simulink model "Copy_of_ModeStatAndRsp"  (R2018b)
settings: Solver=FixedStepDiscrete  StartTime=0.0  StopTime=10.0  FixedStep=0.01  RelTol=1e-3
undefined symbols (not defined in the file): c_RecvL, c_RecvLR, c_RecvR, IfVeSMSeStNumConfig, KeSMSbMdChime2Enable_Val, KeSMSbSRSPosNumConfig_Val, KeSMSuChmReqDurnTm_Val, KeSMSuChmReqIntlTm_Val, KeSMSuRspStatHldTm_Val, MdRspLocal1, MdTp1, ModeNum, PowerMode1, SrcReqTp1, srsconvert
libraries: RspLib x47, simulink x1
(part 4 of 8)

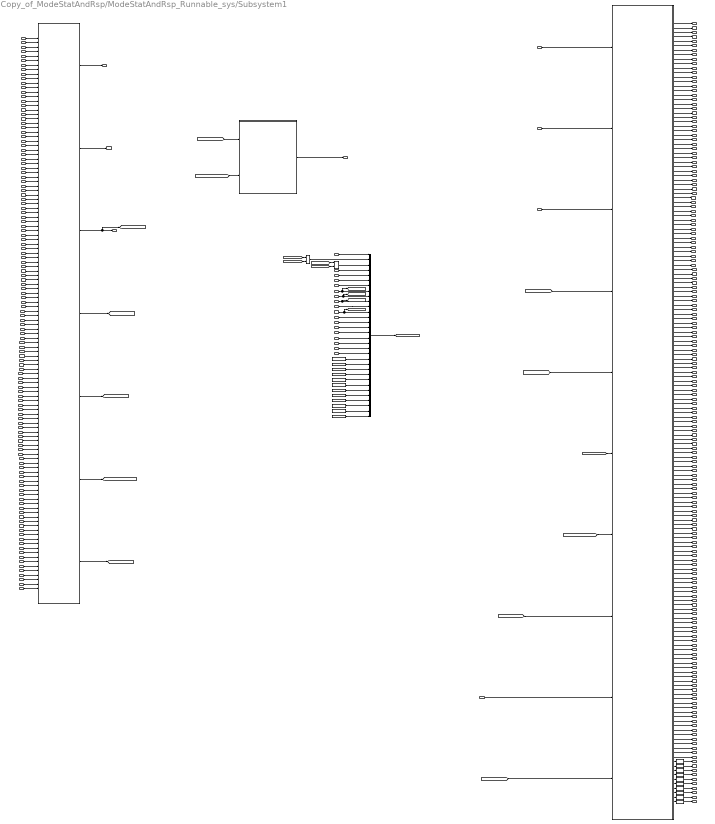
== system Copy_of_ModeStatAndRsp/ModeStatAndRsp_Runnable_sys/Subsystem1 ==
  acsExtMdReq : Inport
  acsEntyMdReq : Inport  Port=2
  LtVipMdReq : Inport  Port=3
  RtVipMdReq : Inport  Port=4
  AllVipMdReq : Inport  Port=5
  LtLugMdReq : Inport  Port=6
  RtLugMdReq : Inport  Port=7
  AllLugMdReq : Inport  Port=8
  LtRcvyMdReq : Inport  Port=9
  RtRcvyMdReq : Inport  Port=10
  CommCond : Inport  Port=11
  CommExitCond : Inport  Port=12
  CommExitCondwithSpeed : Inport  Port=13
  isAcsMdEntryDoneOK : Inport  Port=14
  isAcsMdExtDoneOK : Inport  Port=15
  isLfLugDoneOK : Inport  Port=16
  isLfRecoveryDoneOK : Inport  Port=17
  isLfVipDoneOK : Inport  Port=18
  isRtLugDoneOK : Inport  Port=19
  isRtRecoveryDoneOK : Inport  Port=20
  isRtVipDoneOK : Inport  Port=21
  isAcsMdEntryDoneFailed : Inport  Port=22
  isAcsMdExtDoneFailed : Inport  Port=23
  isLfLugDoneFailed : Inport  Port=24
  isLfRecoveryDoneFailed : Inport  Port=25
  isLfVipDoneFailed : Inport  Port=26
  isRtLugDoneFailed : Inport  Port=27
  isRtRecoveryDoneFailed : Inport  Port=28
  isRtVipDoneFailed : Inport  Port=29
  SwIntAcsEnty : Inport  Port=30
  SwIntAcsExt : Inport  Port=31
  SwIntLfVip : Inport  Port=32
  SwIntRtVip : Inport  Port=33
  SwIntLfLug : Inport  Port=34
  SwIntRtLug : Inport  Port=35
  SwIntLfRcvy : Inport  Port=36
  SwIntRtRcvy : Inport  Port=37
  SwIntAllLug : Inport  Port=38
  SoftIntAcsExt : Inport  Port=39
  SoftIntAcsEnty : Inport  Port=40
  SoftIntLfVip : Inport  Port=41
  SoftIntRtVip : Inport  Port=42
  SoftIntLfLug : Inport  Port=43
  SoftIntRtLug : Inport  Port=44
  SoftIntLfRcvy : Inport  Port=45
  SoftIntRtRcvy : Inport  Port=46
  SoftIntAllVip : Inport  Port=47
  SoftIntAllLug : Inport  Port=48
  acsExtMdSrcTp : Inport  Port=49
  acsEntyMdSrcTp : Inport  Port=50
  LtVipSrcReqTp : Inport  Port=51
  RtVipSrcReqTp : Inport  Port=52
  LtLugSrcReqTp : Inport  Port=53
  RtLugSrcReqTp : Inport  Port=54
  LtRcvySrcReqTp : Inport  Port=55
  RtRcvySrcReqTp : Inport  Port=56
  PwrMdChked : Inport  Port=57
  isLfLugArrivedAtTargetPos : Inport  Port=58
  isRtLugArrivedAtTargetPos : Inport  Port=59
  isLfVipArrivedAtTargetPos : Inport  Port=60
  isRtVipArrivedAtTargetPos : Inport  Port=61
  isAcsMdEntryArrivedAtTargetPos : Inport  Port=62
  isAcsMdExtArrivedAtTargetPos : Inport  Port=63
  isLfRecoveryArrivedAtTargetPos : Inport  Port=64
  isRtRecoveryArrivedAtTargetPos : Inport  Port=65
  IfVeSMSuChmMgrStat_Val_read : Inport  Port=66
  KeSMSuRspStatHldTm_Val : Inport  Port=67
  AllLugSrcReqTp_Val : Inport  Port=68
  StNumConfig : Inport  Port=69
  isAcsMdINTMAtTargetPos : Inport  Port=70
  isAcsMdFamlyLAtTargetPos : Inport  Port=71
  isAcsMdFamlyRAtTargetPos : Inport  Port=72
  isLyLArrivedAtTargetPos : Inport  Port=73
  isLyRArrivedAtTargetPos : Inport  Port=74
  isINTMDoneOK : Inport  Port=75
  isFamlyLDoneOK : Inport  Port=76
  isFamlyRDoneOK : Inport  Port=77
  isLfLyDoneOK : Inport  Port=78
  isRtLyDoneOK : Inport  Port=79
  isINTMDoneFailed : Inport  Port=80
  isFamlyLDoneFailed : Inport  Port=81
  isFamlyRDoneFailed : Inport  Port=82
  isLfLyDoneFailed : Inport  Port=83
  isRtLyDoneFailed : Inport  Port=84
  INTMMdReq_Val_read : Inport  Port=85
  INTMSrcReqTp_Val_read : Inport  Port=86
  LfFamlyReq_Val_read : Inport  Port=87
  LfFamlySrcReqTp_Val_read : Inport  Port=88
  LfLyMdReq_Val_read : Inport  Port=89
  LfLySrcReqTp_Val_read : Inport  Port=90
  RtFamlyMdReq_Val_read : Inport  Port=91
  RtFamlySrcReqTp_Val_read : Inport  Port=92
  RtLyMdReq_Val_read : Inport  Port=93
  RtLySrcReqTp_Val_read : Inport  Port=94
  SoftIntINTM_Val_read : Inport  Port=95
  SoftIntLfFamly_Val_read : Inport  Port=96
  SoftIntLfLy_Val_read : Inport  Port=97
  SoftIntRtFamly_Val_read : Inport  Port=98
  SoftIntRtLy_Val_read : Inport  Port=99
  SwIntINTM_Val_read : Inport  Port=100
  SwIntLfFamly_Val_read : Inport  Port=101
  SwIntLfLy_Val_read : Inport  Port=102
  SwIntRtFamly_Val_read : Inport  Port=103
  SwIntRtLy_Val_read : Inport  Port=104
  PosArray_Val_read : Inport  Port=105
  AllVipSrcReqTp_Val_read : Inport  Port=106
  LugMdLtAvl_Val_read : Inport  Port=107
  LugMdRtAvl_Val_read : Inport  Port=108
  VipMdLtAvl_Val_read : Inport  Port=109
  VipMdRtAvl_Val_read : Inport  Port=110
  SwIntAllVip_Val_read : Inport  Port=111
  IntimacyRtMdReq_Val_read : Inport  Port=112
  IntimacyRtMdSrcTp_Val_read : Inport  Port=113
  isINTMRArrivedAtTargetPos_Val_read : Inport  Port=114
  isINTMRDoneFailed_Val_read : Inport  Port=115
  isINTMRDoneOK_Val_read : Inport  Port=116
  isLgrstCloseLArrivedAtTargetPos_Val_read : Inport  Port=117
  isLgrstCloseLDoneFailed_Val_read : Inport  Port=118
  isLgrstCloseLDoneOK_Val_read : Inport  Port=119
  isLgrstCloseRArrivedAtTargetPos_Val_read : Inport  Port=120
  isLgrstCloseRDoneFailed_Val_read : Inport  Port=121
  isLgrstCloseRDoneOK_Val_read : Inport  Port=122
  isLgrstOpenLArrivedAtTargetPos_Val_read : Inport  Port=123
  isLgrstOpenLDoneFailed_Val_read : Inport  Port=124
  isLgrstOpenLDoneOK_Val_read : Inport  Port=125
  isLgrstOpenRArrivedAtTargetPos_Val_read : Inport  Port=126
  isLgrstOpenRDoneFailed_Val_read : Inport  Port=127
  isLgrstOpenRDoneOK_Val_read : Inport  Port=128
  LgrstCloseLtMdReq_Val_read : Inport  Port=129
  LgrstCloseLtSrcReqTp_Val_read : Inport  Port=130
  LgrstCloseRtMdReq_Val_read : Inport  Port=131
  LgrstCloseRtSrcReqTp_Val_read : Inport  Port=132
  LgrstOpenLtMdReq_Val_read : Inport  Port=133
  LgrstOpenLtSrcReqTp_Val_read : Inport  Port=134
  LgrstOpenRtMdReq_Val_read : Inport  Port=135
  LgrstOpenRtSrcReqTp_Val_read : Inport  Port=136
  SoftIntIntimacyRt_Val_read : Inport  Port=137
  SoftIntLgrstCloseLt_Val_read : Inport  Port=138
  SoftIntLgrstCloseRt_Val_read : Inport  Port=139
  SoftIntLgrstOpenLt_Val_read : Inport  Port=140
  SoftIntLgrstOpenRt_Val_read : Inport  Port=141
  SwIntIntimacyRt_Val_read : Inport  Port=142
  SwIntLgrstCloseLt_Val_read : Inport  Port=143
  SwIntLgrstCloseRt_Val_read : Inport  Port=144
  SwIntLgrstOpenLt_Val_read : Inport  Port=145
  SwIntLgrstOpenRt_Val_read : Inport  Port=146
  AND : Logic  AllPortsSameDT=off  OutDataTypeStr=boolean
  AND1 : Logic  AllPortsSameDT=off  OutDataTypeStr=boolean
  Bus Creator2 : BusCreator  Inputs=32
  Constant{39..50} (12 alike) : Constant  Value=0  OutDataTypeStr=boolean
  Data Type Conversion{,1..9} (10 alike) : DataTypeConversion  OutDataTypeStr=uint8
  FeedbackModeStatAndRsp : Subsystem
  SRSModeCheck : Subsystem
  Subsystem : Subsystem
  oModeState : Outport
  IfVeSMSeStPassCmprtMdCrtMdStat_Val_write : Outport  Port=2
  IfVeSMSeStPassCmprtMdHMIDisCmdSrv_Val_write : Outport  Port=3  VectorParamsAs1DForOutWhenUnconnected=on
  ModeSrcTpLt : Outport  Port=4  VectorParamsAs1DForOutWhenUnconnected=on
  IfVeSMSeStPassCmprtMdNoti2ChmEvntStat_Val_write : Outport  Port=5  VectorParamsAs1DForOutWhenUnconnected=on
  SRSCrtMdIndTyp_67_2_Val_write : Outport  Port=6  VectorParamsAs1DForOutWhenUnconnected=on
  ModeState32 : Outport  Port=7  VectorParamsAs1DForOutWhenUnconnected=on
  SRSMode : Outport  Port=8  VectorParamsAs1DForOutWhenUnconnected=on
  StPassCmprtMd1RclRspStat : Outport  Port=9  VectorParamsAs1DForOutWhenUnconnected=on
  StPassCmprtMd2RclRspStat : Outport  Port=10  VectorParamsAs1DForOutWhenUnconnected=on
  StPassCmprtMd3RclRspStat : Outport  Port=11  VectorParamsAs1DForOutWhenUnconnected=on
  StPassCmprtMd4RclRspStat : Outport  Port=12  VectorParamsAs1DForOutWhenUnconnected=on
  StPassCmprtMd5RclRspStat : Outport  Port=13  VectorParamsAs1DForOutWhenUnconnected=on
  StPassCmprtMd6RclRspStat : Outport  Port=14  VectorParamsAs1DForOutWhenUnconnected=on
  StPassCmprtMd7RclRspStat : Outport  Port=15  VectorParamsAs1DForOutWhenUnconnected=on
  StPassCmprtMd8RclRspStat : Outport  Port=16  VectorParamsAs1DForOutWhenUnconnected=on
  StPassCmprtMd9RclRspStat : Outport  Port=17  VectorParamsAs1DForOutWhenUnconnected=on
  StPassCmprtMd10RclRspStat : Outport  Port=18  VectorParamsAs1DForOutWhenUnconnected=on
  StPassCmprtMd11RclRspStat : Outport  Port=19  VectorParamsAs1DForOutWhenUnconnected=on
  StPassCmprtMd12RclRspStat : Outport  Port=20  VectorParamsAs1DForOutWhenUnconnected=on
  StPassCmprtMd13RclRspStat : Outport  Port=21  VectorParamsAs1DForOutWhenUnconnected=on
  StPassCmprtMd14RclRspStat : Outport  Port=22  VectorParamsAs1DForOutWhenUnconnected=on
  StPassCmprtMd15RclRspStat : Outport  Port=23  VectorParamsAs1DForOutWhenUnconnected=on
  StPassCmprtMd16RclRspStat : Outport  Port=24  VectorParamsAs1DForOutWhenUnconnected=on
  StPassCmprtMd17RclRspStat : Outport  Port=25  VectorParamsAs1DForOutWhenUnconnected=on
  StPassCmprtMd18RclRspStat : Outport  Port=26  VectorParamsAs1DForOutWhenUnconnected=on
  StPassCmprtMd19RclRspStat : Outport  Port=27  VectorParamsAs1DForOutWhenUnconnected=on
  StPassCmprtMd20RclRspStat : Outport  Port=28  VectorParamsAs1DForOutWhenUnconnected=on
  StPassCmprtMd21RclRspStat : Outport  Port=29  VectorParamsAs1DForOutWhenUnconnected=on
  StPassCmprtMd22RclRspStat : Outport  Port=30  VectorParamsAs1DForOutWhenUnconnected=on
  StPassCmprtMd23RclRspStat : Outport  Port=31  VectorParamsAs1DForOutWhenUnconnected=on
  StPassCmprtMd24RclRspStat : Outport  Port=32  VectorParamsAs1DForOutWhenUnconnected=on
  StPassCmprtMd25RclRspStat : Outport  Port=33  VectorParamsAs1DForOutWhenUnconnected=on
  StPassCmprtMd26RclRspStat : Outport  Port=34  VectorParamsAs1DForOutWhenUnconnected=on
  StPassCmprtMd27RclRspStat : Outport  Port=35  VectorParamsAs1DForOutWhenUnconnected=on
  StPassCmprtMd28RclRspStat : Outport  Port=36  VectorParamsAs1DForOutWhenUnconnected=on
  StPassCmprtMd29RclRspStat : Outport  Port=37  VectorParamsAs1DForOutWhenUnconnected=on
  StPassCmprtMd30RclRspStat : Outport  Port=38  VectorParamsAs1DForOutWhenUnconnected=on
  StPassCmprtMd31RclRspStat : Outport  Port=39  VectorParamsAs1DForOutWhenUnconnected=on
  StPassCmprtMd32RclRspStat : Outport  Port=40  VectorParamsAs1DForOutWhenUnconnected=on
  StPassCmprtMd_RfCtrl_Sw_RclRspStat : Outport  Port=41  VectorParamsAs1DForOutWhenUnconnected=on
  StSrv_StMd1_Rsp : Outport  Port=42  VectorParamsAs1DForOutWhenUnconnected=on
  StSrv_StMd2_Rsp : Outport  Port=43  VectorParamsAs1DForOutWhenUnconnected=on
  StSrv_StMd3_Rsp : Outport  Port=44  VectorParamsAs1DForOutWhenUnconnected=on
  StSrv_StMd4_Rsp : Outport  Port=45  VectorParamsAs1DForOutWhenUnconnected=on
  StSrv_StMd5_Rsp : Outport  Port=46  VectorParamsAs1DForOutWhenUnconnected=on
  StSrv_StMd6_Rsp : Outport  Port=47  VectorParamsAs1DForOutWhenUnconnected=on
  StSrv_StMd7_Rsp : Outport  Port=48  VectorParamsAs1DForOutWhenUnconnected=on
  StSrv_StMd8_Rsp : Outport  Port=49  VectorParamsAs1DForOutWhenUnconnected=on
  StSrv_StMd9_Rsp : Outport  Port=50  VectorParamsAs1DForOutWhenUnconnected=on
  StSrv_StMd10_Rsp : Outport  Port=51  VectorParamsAs1DForOutWhenUnconnected=on
  StSrv_StMd11_Rsp : Outport  Port=52  VectorParamsAs1DForOutWhenUnconnected=on
  StSrv_StMd12_Rsp : Outport  Port=53  VectorParamsAs1DForOutWhenUnconnected=on
  StSrv_StMd13_Rsp : Outport  Port=54  VectorParamsAs1DForOutWhenUnconnected=on
  StSrv_StMd14_Rsp : Outport  Port=55  VectorParamsAs1DForOutWhenUnconnected=on
  StSrv_StMd15_Rsp : Outport  Port=56  VectorParamsAs1DForOutWhenUnconnected=on
  StSrv_StMd16_Rsp : Outport  Port=57  VectorParamsAs1DForOutWhenUnconnected=on
  StSrv_StMd17_Rsp : Outport  Port=58  VectorParamsAs1DForOutWhenUnconnected=on
  StSrv_StMd18_Rsp : Outport  Port=59  VectorParamsAs1DForOutWhenUnconnected=on
  StSrv_StMd19_Rsp : Outport  Port=60  VectorParamsAs1DForOutWhenUnconnected=on
  StSrv_StMd20_Rsp : Outport  Port=61  VectorParamsAs1DForOutWhenUnconnected=on
  StSrv_StMd21_Rsp : Outport  Port=62  VectorParamsAs1DForOutWhenUnconnected=on
  StSrv_StMd22_Rsp : Outport  Port=63  VectorParamsAs1DForOutWhenUnconnected=on
  StSrv_StMd23_Rsp : Outport  Port=64  VectorParamsAs1DForOutWhenUnconnected=on
  StSrv_StMd24_Rsp : Outport  Port=65  VectorParamsAs1DForOutWhenUnconnected=on
  StSrv_StMd25_Rsp : Outport  Port=66  VectorParamsAs1DForOutWhenUnconnected=on
  StSrv_StMd26_Rsp : Outport  Port=67  VectorParamsAs1DForOutWhenUnconnected=on
  StSrv_StMd27_Rsp : Outport  Port=68  VectorParamsAs1DForOutWhenUnconnected=on
  StSrv_StMd28_Rsp : Outport  Port=69  VectorParamsAs1DForOutWhenUnconnected=on
  StSrv_StMd29_Rsp : Outport  Port=70  VectorParamsAs1DForOutWhenUnconnected=on
  StSrv_StMd30_Rsp : Outport  Port=71  VectorParamsAs1DForOutWhenUnconnected=on
  StSrv_StMd31_Rsp : Outport  Port=72  VectorParamsAs1DForOutWhenUnconnected=on
  StSrv_StMd32_Rsp : Outport  Port=73  VectorParamsAs1DForOutWhenUnconnected=on
  HMI_2L_StMd1_Rsp : Outport  Port=74  VectorParamsAs1DForOutWhenUnconnected=on
  HMI_2L_StMd2_Rsp : Outport  Port=75  VectorParamsAs1DForOutWhenUnconnected=on
  HMI_2L_StMd3_Rsp : Outport  Port=76  VectorParamsAs1DForOutWhenUnconnected=on
  HMI_2L_StMd4_Rsp : Outport  Port=77  VectorParamsAs1DForOutWhenUnconnected=on
  HMI_2L_StMd5_Rsp : Outport  Port=78  VectorParamsAs1DForOutWhenUnconnected=on
  HMI_2L_StMd6_Rsp : Outport  Port=79  VectorParamsAs1DForOutWhenUnconnected=on
  HMI_2L_StMd7_Rsp : Outport  Port=80  VectorParamsAs1DForOutWhenUnconnected=on
  HMI_2L_StMd8_Rsp : Outport  Port=81  VectorParamsAs1DForOutWhenUnconnected=on
  HMI_2L_StMd9_Rsp : Outport  Port=82  VectorParamsAs1DForOutWhenUnconnected=on
  HMI_2L_StMd10_Rsp : Outport  Port=83  VectorParamsAs1DForOutWhenUnconnected=on
  HMI_2L_StMd11_Rsp : Outport  Port=84  VectorParamsAs1DForOutWhenUnconnected=on
  HMI_2L_StMd12_Rsp : Outport  Port=85  VectorParamsAs1DForOutWhenUnconnected=on
  HMI_2L_StMd13_Rsp : Outport  Port=86  VectorParamsAs1DForOutWhenUnconnected=on
  HMI_2L_StMd14_Rsp : Outport  Port=87  VectorParamsAs1DForOutWhenUnconnected=on
  HMI_2L_StMd15_Rsp : Outport  Port=88  VectorParamsAs1DForOutWhenUnconnected=on
  HMI_2L_StMd16_Rsp : Outport  Port=89  VectorParamsAs1DForOutWhenUnconnected=on
  HMI_2L_StMd17_Rsp : Outport  Port=90  VectorParamsAs1DForOutWhenUnconnected=on
  HMI_2L_StMd18_Rsp : Outport  Port=91  VectorParamsAs1DForOutWhenUnconnected=on
  HMI_2L_StMd19_Rsp : Outport  Port=92  VectorParamsAs1DForOutWhenUnconnected=on
  HMI_2L_StMd20_Rsp : Outport  Port=93  VectorParamsAs1DForOutWhenUnconnected=on
  HMI_2L_StMd21_Rsp : Outport  Port=94  VectorParamsAs1DForOutWhenUnconnected=on
  HMI_2L_StMd22_Rsp : Outport  Port=95  VectorParamsAs1DForOutWhenUnconnected=on
  HMI_2L_StMd23_Rsp : Outport  Port=96  VectorParamsAs1DForOutWhenUnconnected=on
  HMI_2L_StMd24_Rsp : Outport  Port=97  VectorParamsAs1DForOutWhenUnconnected=on
  HMI_2L_StMd25_Rsp : Outport  Port=98  VectorParamsAs1DForOutWhenUnconnected=on
  HMI_2L_StMd26_Rsp : Outport  Port=99  VectorParamsAs1DForOutWhenUnconnected=on
  HMI_2L_StMd27_Rsp : Outport  Port=100  VectorParamsAs1DForOutWhenUnconnected=on
  HMI_2L_StMd28_Rsp : Outport  Port=101  VectorParamsAs1DForOutWhenUnconnected=on
  HMI_2L_StMd29_Rsp : Outport  Port=102  VectorParamsAs1DForOutWhenUnconnected=on
  HMI_2L_StMd30_Rsp : Outport  Port=103  VectorParamsAs1DForOutWhenUnconnected=on
  HMI_2L_StMd31_Rsp : Outport  Port=104  VectorParamsAs1DForOutWhenUnconnected=on
  HMI_2L_StMd32_Rsp : Outport  Port=105  VectorParamsAs1DForOutWhenUnconnected=on
  HMI_2R_StMd1_Rsp : Outport  Port=106  VectorParamsAs1DForOutWhenUnconnected=on
  HMI_2R_StMd2_Rsp : Outport  Port=107  VectorParamsAs1DForOutWhenUnconnected=on
  HMI_2R_StMd3_Rsp : Outport  Port=108  VectorParamsAs1DForOutWhenUnconnected=on
  HMI_2R_StMd4_Rsp : Outport  Port=109  VectorParamsAs1DForOutWhenUnconnected=on
  HMI_2R_StMd5_Rsp : Outport  Port=110  VectorParamsAs1DForOutWhenUnconnected=on
  HMI_2R_StMd6_Rsp : Outport  Port=111  VectorParamsAs1DForOutWhenUnconnected=on
  HMI_2R_StMd7_Rsp : Outport  Port=112  VectorParamsAs1DForOutWhenUnconnected=on
  HMI_2R_StMd8_Rsp : Outport  Port=113  VectorParamsAs1DForOutWhenUnconnected=on
  HMI_2R_StMd9_Rsp : Outport  Port=114  VectorParamsAs1DForOutWhenUnconnected=on
  HMI_2R_StMd10_Rsp : Outport  Port=115  VectorParamsAs1DForOutWhenUnconnected=on
  HMI_2R_StMd11_Rsp : Outport  Port=116  VectorParamsAs1DForOutWhenUnconnected=on
  HMI_2R_StMd12_Rsp : Outport  Port=117  VectorParamsAs1DForOutWhenUnconnected=on
  HMI_2R_StMd13_Rsp : Outport  Port=118  VectorParamsAs1DForOutWhenUnconnected=on
  HMI_2R_StMd14_Rsp : Outport  Port=119  VectorParamsAs1DForOutWhenUnconnected=on
  HMI_2R_StMd15_Rsp : Outport  Port=120  VectorParamsAs1DForOutWhenUnconnected=on
  HMI_2R_StMd16_Rsp : Outport  Port=121  VectorParamsAs1DForOutWhenUnconnected=on
  HMI_2R_StMd17_Rsp : Outport  Port=122  VectorParamsAs1DForOutWhenUnconnected=on
  HMI_2R_StMd18_Rsp : Outport  Port=123  VectorParamsAs1DForOutWhenUnconnected=on
  HMI_2R_StMd19_Rsp : Outport  Port=124  VectorParamsAs1DForOutWhenUnconnected=on
  HMI_2R_StMd20_Rsp : Outport  Port=125  VectorParamsAs1DForOutWhenUnconnected=on
  HMI_2R_StMd21_Rsp : Outport  Port=126  VectorParamsAs1DForOutWhenUnconnected=on
  HMI_2R_StMd22_Rsp : Outport  Port=127  VectorParamsAs1DForOutWhenUnconnected=on
  HMI_2R_StMd23_Rsp : Outport  Port=128  VectorParamsAs1DForOutWhenUnconnected=on
  HMI_2R_StMd24_Rsp : Outport  Port=129  VectorParamsAs1DForOutWhenUnconnected=on
  HMI_2R_StMd25_Rsp : Outport  Port=130  VectorParamsAs1DForOutWhenUnconnected=on
  HMI_2R_StMd26_Rsp : Outport  Port=131  VectorParamsAs1DForOutWhenUnconnected=on
  HMI_2R_StMd27_Rsp : Outport  Port=132  VectorParamsAs1DForOutWhenUnconnected=on
  HMI_2R_StMd28_Rsp : Outport  Port=133  VectorParamsAs1DForOutWhenUnconnected=on
  HMI_2R_StMd29_Rsp : Outport  Port=134  VectorParamsAs1DForOutWhenUnconnected=on
  HMI_2R_StMd30_Rsp : Outport  Port=135  VectorParamsAs1DForOutWhenUnconnected=on
  HMI_2R_StMd31_Rsp : Outport  Port=136  VectorParamsAs1DForOutWhenUnconnected=on
  HMI_2R_StMd32_Rsp : Outport  Port=137  VectorParamsAs1DForOutWhenUnconnected=on
  StPassCmprtMd_Md1_CrtStat : Outport  Port=138
  StPassCmprtMd_Md2_CrtStat : Outport  Port=139
  StPassCmprtMd_Md3_CrtStat : Outport  Port=140
  StPassCmprtMd_Md4_CrtStat : Outport  Port=141
  StPassCmprtMd_Md5_CrtStat : Outport  Port=142
  StPassCmprtMd_Md6_CrtStat : Outport  Port=143
  StPassCmprtMd_Md7_CrtStat : Outport  Port=144
  StPassCmprtMd_Md8_CrtStat : Outport  Port=145
  StPassCmprtMd_Md9_CrtStat : Outport  Port=146
  StPassCmprtMd_Md10_CrtStat : Outport  Port=147
  StPassCmprtMd_Md11_CrtStat : Outport  Port=148
  StPassCmprtMd_Md12_CrtStat : Outport  Port=149
  StPassCmprtMd_Md13_CrtStat : Outport  Port=150
  StPassCmprtMd_Md14_CrtStat : Outport  Port=151
  StPassCmprtMd_Md15_CrtStat : Outport  Port=152
  StPassCmprtMd_Md16_CrtStat : Outport  Port=153
  StPassCmprtMd_Md17_CrtStat : Outport  Port=154
  StPassCmprtMd_Md18_CrtStat : Outport  Port=155
  StPassCmprtMd_Md19_CrtStat : Outport  Port=156
  StPassCmprtMd_Md20_CrtStat : Outport  Port=157
  StPassCmprtMd_Md21_CrtStat : Outport  Port=158
  StPassCmprtMd_Md22_CrtStat : Outport  Port=159
  StPassCmprtMd_Md23_CrtStat : Outport  Port=160
  StPassCmprtMd_Md24_CrtStat : Outport  Port=161
  StPassCmprtMd_Md25_CrtStat : Outport  Port=162
  StPassCmprtMd_Md26_CrtStat : Outport  Port=163
  StPassCmprtMd_Md27_CrtStat : Outport  Port=164
  StPassCmprtMd_Md28_CrtStat : Outport  Port=165
  StPassCmprtMd_Md29_CrtStat : Outport  Port=166
  StPassCmprtMd_Md30_CrtStat : Outport  Port=167
  StPassCmprtMd_Md31_CrtStat : Outport  Port=168
  StPassCmprtMd_Md32_CrtStat : Outport  Port=169
  SRSCrt_MdSw1_Stat_67_2 : Outport  Port=170
  SRSCrt_MdSw2_Stat_67_2 : Outport  Port=171
  SRSCrt_MdSw3_Stat_67_2 : Outport  Port=172
  SRSCrt_MdSw4_Stat_67_2 : Outport  Port=173
  SRSCrt_MdSw5_Stat_67_2 : Outport  Port=174
  SRSCrt_MdSw6_Stat_67_2 : Outport  Port=175
  SRSCrt_MdSw7_Stat_67_2 : Outport  Port=176
  SRSCrt_MdSw8_Stat_67_2 : Outport  Port=177
  SRSCrt_MdSw9_Stat_67_2 : Outport  Port=178
  SRSCrt_MdSw10_Stat_67_2 : Outport  Port=179
  wires:
  isLfRecoveryDoneOK/1 -> Subsystem/17(isLfRecoveryDoneOK)
  SwIntAcsExt/1 -> Subsystem/31(SwIntAcsExt)
  SwIntRtVip/1 -> Subsystem/33(SwIntRtVip)
  CommExitCond/1 -> Subsystem/12(CommExitCond)
  isLfVipDoneFailed/1 -> Subsystem/26(isLfVipDoneFailed)
  PwrMdChked/1 -> FeedbackModeStatAndRsp/2(PwrMdChked)
  SoftIntAcsEnty/1 -> Subsystem/40(SoftIntAcsEnty)
  SoftIntRtRcvy/1 -> Subsystem/46(SoftIntRtRcvy)
  SoftIntAllVip/1 -> Subsystem/47(SoftIntAllVip)
  SoftIntLfLug/1 -> Subsystem/43(SoftIntLfLug)
  FeedbackModeStatAndRsp/1(StPassCmprtMdHMIDisCmd) -> IfVeSMSeStPassCmprtMdHMIDisCmdSrv_Val_write/1
  SwIntAcsEnty/1 -> Subsystem/30(SwIntAcsEnty)
  isAcsMdEntryDoneFailed/1 -> Subsystem/22(isAcsMdEntryDoneFailed)
  isRtVipDoneFailed/1 -> Subsystem/29(isRtVipDoneFailed)
  SoftIntRtLug/1 -> Subsystem/44(SoftIntRtLug)
  FeedbackModeStatAndRsp/4(StPassCmprtMdCrtMdStat) -> IfVeSMSeStPassCmprtMdCrtMdStat_Val_write/1
  isRtRecoveryDoneFailed/1 -> Subsystem/28(isRtRecoveryDoneFailed)
  KeSMSuRspStatHldTm_Val/1 -> FeedbackModeStatAndRsp/1(rspStateHldTm)
  isLfRecoveryDoneFailed/1 -> Subsystem/25(isLfRecoveryDoneFailed)
  isAcsMdExtDoneOK/1 -> Subsystem/15(isAcsMdExtDoneOK)
  isRtLugDoneOK/1 -> Subsystem/19(isRtLugDoneOK)
  SwIntRtRcvy/1 -> Subsystem/37(SwIntRtRcvy)
  SwIntLfLug/1 -> Subsystem/34(SwIntLfLug)
  SwIntLfRcvy/1 -> Subsystem/36(SwIntLfRcvy)
  CommCond/1 -> Subsystem/11(CommCond)
  SoftIntAllLug/1 -> Subsystem/48(SoftIntAllLug)
  SwIntAllLug/1 -> Subsystem/38(SwIntAllLug)
  isLfLugDoneFailed/1 -> Subsystem/24(isLfLugDoneFailed)
  SoftIntRtVip/1 -> Subsystem/42(SoftIntRtVip)
  SwIntLfVip/1 -> Subsystem/32(SwIntLfVip)
  FeedbackModeStatAndRsp/2(IfVeSMSeStPassCmprtMdNoti2ChmEvntStat_Val_write) -> IfVeSMSeStPassCmprtMdNoti2ChmEvntStat_Val_write/1
  Subsystem/1(oModeState) -> oModeState/1
  SoftIntAcsExt/1 -> Subsystem/39(SoftIntAcsExt)
  isAcsMdExtDoneFailed/1 -> Subsystem/23(isAcsMdExtDoneFailed)
  SoftIntLfVip/1 -> Subsystem/41(SoftIntLfVip)
  isAcsMdEntryDoneOK/1 -> Subsystem/14(isAcsMdEntryDoneOK)
  isRtRecoveryDoneOK/1 -> Subsystem/20(isRtRecoveryDoneOK)
  isLfVipDoneOK/1 -> Subsystem/18(isLfVipDoneOK)
  isRtVipDoneOK/1 -> Subsystem/21(isRtVipDoneOK)
  CommExitCondwithSpeed/1 -> Subsystem/13(CommExitCondwithSpeed)
  isLfLugDoneOK/1 -> Subsystem/16(isLfLugDoneOK)
  SoftIntLfRcvy/1 -> Subsystem/45(SoftIntLfRcvy)
  IfVeSMSuChmMgrStat_Val_read/1 -> FeedbackModeStatAndRsp/3(ChmMgrStat)
  isRtLugDoneFailed/1 -> Subsystem/27(isRtLugDoneFailed)
  SwIntRtLug/1 -> Subsystem/35(SwIntRtLug)
  FeedbackModeStatAndRsp/3(SRSCrtMdIndTyp_67_2_Val_write) -> SRSCrtMdIndTyp_67_2_Val_write/1
  Subsystem/2(ModeSrcTpLt) -> ModeSrcTpLt/1
  Subsystem/3(ModeState32) -> ModeState32/1, [ModeState32]
  [ModeState32] -> FeedbackModeStatAndRsp/4(ModeState32)
  acsExtMdReq/1 -> Subsystem/1(acsExtMdReq)
  acsEntyMdReq/1 -> Subsystem/2(acsEntyMdReq)
  LtVipMdReq/1 -> Subsystem/3(LtVipMdReq)
  RtVipMdReq/1 -> Subsystem/4(RtVipMdReq)
  AllVipMdReq/1 -> Subsystem/5(AllVipMdReq)
  LtLugMdReq/1 -> Subsystem/6(LtLugMdReq)
  RtLugMdReq/1 -> Subsystem/7(RtLugMdReq)
  AllLugMdReq/1 -> Subsystem/8(AllLugMdReq)
  LtRcvyMdReq/1 -> Subsystem/9(LtRcvyMdReq)
  RtRcvyMdReq/1 -> Subsystem/10(RtRcvyMdReq)
  acsExtMdSrcTp/1 -> Subsystem/49(acsExtMdSrcTp)
  acsEntyMdSrcTp/1 -> Subsystem/50(acsEntyMdSrcTp)
  LtVipSrcReqTp/1 -> Subsystem/51(LtVipSrcReqTp)
  RtVipSrcReqTp/1 -> Subsystem/52(RtVipSrcReqTp)
  LtLugSrcReqTp/1 -> Subsystem/53(LtLugSrcReqTp)
  RtLugSrcReqTp/1 -> Subsystem/54(RtLugSrcReqTp)
  LtRcvySrcReqTp/1 -> Subsystem/55(LtRcvySrcReqTp)
  RtRcvySrcReqTp/1 -> Subsystem/56(RtRcvySrcReqTp)
  AllLugSrcReqTp_Val/1 -> Subsystem/57(AllLugSrcReqTp_Val)
  StNumConfig/1 -> Subsystem/58(StNumConfig)
  [MdStateBus] -> FeedbackModeStatAndRsp/5(ModeStateBus)
  Bus Creator2/1 -> [MdTrgtPos]  "TrgtPos"
  isAcsMdEntryArrivedAtTargetPos/1 -> Bus Creator2/1  "Md1TrgtPos"
  isAcsMdExtArrivedAtTargetPos/1 -> Bus Creator2/4  "Md4TrgtPos"
  isAcsMdINTMAtTargetPos/1 -> Bus Creator2/5  "Md5TrgtPos"
  isAcsMdFamlyRAtTargetPos/1 -> Bus Creator2/6  "Md6TrgtPos"
  isAcsMdFamlyLAtTargetPos/1 -> Bus Creator2/7  "Md7TrgtPos"
  isLfLugArrivedAtTargetPos/1 -> [isLfLugArrivedAtTargetPos], Bus Creator2/8  "Md8TrgtPos"
  isRtLugArrivedAtTargetPos/1 -> [isRtLugArrivedAtTargetPos], Bus Creator2/9  "Md9TrgtPos"
  isLfVipArrivedAtTargetPos/1 -> [LfVipArrivedAtTargetPos], Bus Creator2/10  "Md10TrgtPos"
  isLfRecoveryArrivedAtTargetPos/1 -> Bus Creator2/11  "Md11TrgtPos"
  isRtVipArrivedAtTargetPos/1 -> [RtVipArrivedAtTargetPos], Bus Creator2/12  "Md12TrgtPos"
  isRtRecoveryArrivedAtTargetPos/1 -> Bus Creator2/13  "Md13TrgtPos"
  isLyLArrivedAtTargetPos/1 -> Bus Creator2/14  "Md14TrgtPos"
  isLyRArrivedAtTargetPos/1 -> Bus Creator2/15  "Md15TrgtPos"
  AND/1 -> Bus Creator2/2  "Md2TrgtPos"
  AND1/1 -> Bus Creator2/3  "Md3TrgtPos"
  isLgrstOpenLArrivedAtTargetPos_Val_read/1 -> Bus Creator2/16  "Md16TrgtPos"
  isLgrstCloseLArrivedAtTargetPos_Val_read/1 -> Bus Creator2/17  "Md17TrgtPos"
  isLgrstOpenRArrivedAtTargetPos_Val_read/1 -> Bus Creator2/18  "Md18TrgtPos"
  isLgrstCloseRArrivedAtTargetPos_Val_read/1 -> Bus Creator2/19  "Md19TrgtPos"
  isINTMRArrivedAtTargetPos_Val_read/1 -> Bus Creator2/20  "Md20TrgtPos"
  Constant39/1 -> Bus Creator2/21  "Md21TrgtPos"
  Constant40/1 -> Bus Creator2/22  "Md22TrgtPos"
  Constant41/1 -> Bus Creator2/23  "Md23TrgtPos"
  Constant42/1 -> Bus Creator2/24  "Md24TrgtPos"
  Constant43/1 -> Bus Creator2/25  "Md25TrgtPos"
  Constant44/1 -> Bus Creator2/26  "Md26TrgtPos"
  Constant45/1 -> Bus Creator2/27  "Md27TrgtPos"
  Constant46/1 -> Bus Creator2/28  "Md28TrgtPos"
  Constant47/1 -> Bus Creator2/29  "Md29TrgtPos"
  Constant48/1 -> Bus Creator2/30  "Md30TrgtPos"
  Constant49/1 -> Bus Creator2/31  "Md31TrgtPos"
  Constant50/1 -> Bus Creator2/32  "Md32TrgtPos"
  FeedbackModeStatAndRsp/9(StPassCmprtMd5RclRspStat) -> StPassCmprtMd5RclRspStat/1
  FeedbackModeStatAndRsp/10(StPassCmprtMd6RclRspStat) -> StPassCmprtMd6RclRspStat/1
  FeedbackModeStatAndRsp/6(StPassCmprtMd2RclRspStat) -> StPassCmprtMd2RclRspStat/1
  FeedbackModeStatAndRsp/5(StPassCmprtMd1RclRspStat) -> StPassCmprtMd1RclRspStat/1
  FeedbackModeStatAndRsp/7(StPassCmprtMd3RclRspStat) -> StPassCmprtMd3RclRspStat/1
  FeedbackModeStatAndRsp/8(StPassCmprtMd4RclRspStat) -> StPassCmprtMd4RclRspStat/1
  FeedbackModeStatAndRsp/11(StPassCmprtMd7RclRspStat) -> StPassCmprtMd7RclRspStat/1
  FeedbackModeStatAndRsp/12(StPassCmprtMd8RclRspStat) -> StPassCmprtMd8RclRspStat/1
  FeedbackModeStatAndRsp/13(StPassCmprtMd9RclRspStat) -> StPassCmprtMd9RclRspStat/1
  FeedbackModeStatAndRsp/14(StPassCmprtMd10RclRspStat) -> StPassCmprtMd10RclRspStat/1
  FeedbackModeStatAndRsp/15(StPassCmprtMd11RclRspStat) -> StPassCmprtMd11RclRspStat/1
  FeedbackModeStatAndRsp/16(StPassCmprtMd12RclRspStat) -> StPassCmprtMd12RclRspStat/1
  FeedbackModeStatAndRsp/17(StPassCmprtMd13RclRspStat) -> StPassCmprtMd13RclRspStat/1
  FeedbackModeStatAndRsp/18(StPassCmprtMd14RclRspStat) -> StPassCmprtMd14RclRspStat/1
  FeedbackModeStatAndRsp/19(StPassCmprtMd15RclRspStat) -> StPassCmprtMd15RclRspStat/1
  FeedbackModeStatAndRsp/20(StPassCmprtMd16RclRspStat) -> StPassCmprtMd16RclRspStat/1
  FeedbackModeStatAndRsp/21(StPassCmprtMd17RclRspStat) -> StPassCmprtMd17RclRspStat/1
  FeedbackModeStatAndRsp/22(StPassCmprtMd18RclRspStat) -> StPassCmprtMd18RclRspStat/1
  FeedbackModeStatAndRsp/23(StPassCmprtMd19RclRspStat) -> StPassCmprtMd19RclRspStat/1
  FeedbackModeStatAndRsp/24(StPassCmprtMd20RclRspStat) -> StPassCmprtMd20RclRspStat/1
  FeedbackModeStatAndRsp/25(StPassCmprtMd21RclRspStat) -> StPassCmprtMd21RclRspStat/1
  FeedbackModeStatAndRsp/26(StPassCmprtMd22RclRspStat) -> StPassCmprtMd22RclRspStat/1
  FeedbackModeStatAndRsp/27(StPassCmprtMd23RclRspStat) -> StPassCmprtMd23RclRspStat/1
  FeedbackModeStatAndRsp/28(StPassCmprtMd24RclRspStat) -> StPassCmprtMd24RclRspStat/1
  FeedbackModeStatAndRsp/29(StPassCmprtMd25RclRspStat) -> StPassCmprtMd25RclRspStat/1
  FeedbackModeStatAndRsp/30(StPassCmprtMd26RclRspStat) -> StPassCmprtMd26RclRspStat/1
  FeedbackModeStatAndRsp/31(StPassCmprtMd27RclRspStat) -> StPassCmprtMd27RclRspStat/1
  FeedbackModeStatAndRsp/32(StPassCmprtMd28RclRspStat) -> StPassCmprtMd28RclRspStat/1
  FeedbackModeStatAndRsp/33(StPassCmprtMd29RclRspStat) -> StPassCmprtMd29RclRspStat/1
  FeedbackModeStatAndRsp/34(StPassCmprtMd30RclRspStat) -> StPassCmprtMd30RclRspStat/1
  FeedbackModeStatAndRsp/35(StPassCmprtMd31RclRspStat) -> StPassCmprtMd31RclRspStat/1
  FeedbackModeStatAndRsp/36(StPassCmprtMd32RclRspStat) -> StPassCmprtMd32RclRspStat/1
  FeedbackModeStatAndRsp/37(StPassCmprtMd_RfCtrl_Sw_RclRspStat) -> StPassCmprtMd_RfCtrl_Sw_RclRspStat/1
  FeedbackModeStatAndRsp/38(StSrv_StMd1_Rsp) -> StSrv_StMd1_Rsp/1
  FeedbackModeStatAndRsp/39(StSrv_StMd2_Rsp) -> StSrv_StMd2_Rsp/1
  FeedbackModeStatAndRsp/40(StSrv_StMd3_Rsp) -> StSrv_StMd3_Rsp/1
  FeedbackModeStatAndRsp/41(StSrv_StMd4_Rsp) -> StSrv_StMd4_Rsp/1
  FeedbackModeStatAndRsp/42(StSrv_StMd5_Rsp) -> StSrv_StMd5_Rsp/1
  FeedbackModeStatAndRsp/43(StSrv_StMd6_Rsp) -> StSrv_StMd6_Rsp/1
  FeedbackModeStatAndRsp/44(StSrv_StMd7_Rsp) -> StSrv_StMd7_Rsp/1
  FeedbackModeStatAndRsp/45(StSrv_StMd8_Rsp) -> StSrv_StMd8_Rsp/1
  FeedbackModeStatAndRsp/46(StSrv_StMd9_Rsp) -> StSrv_StMd9_Rsp/1
  FeedbackModeStatAndRsp/47(StSrv_StMd10_Rsp) -> StSrv_StMd10_Rsp/1
  FeedbackModeStatAndRsp/48(StSrv_StMd11_Rsp) -> StSrv_StMd11_Rsp/1
  FeedbackModeStatAndRsp/49(StSrv_StMd12_Rsp) -> StSrv_StMd12_Rsp/1
  FeedbackModeStatAndRsp/50(StSrv_StMd13_Rsp) -> StSrv_StMd13_Rsp/1
  FeedbackModeStatAndRsp/51(StSrv_StMd14_Rsp) -> StSrv_StMd14_Rsp/1
  FeedbackModeStatAndRsp/52(StSrv_StMd15_Rsp) -> StSrv_StMd15_Rsp/1
  FeedbackModeStatAndRsp/53(StSrv_StMd16_Rsp) -> StSrv_StMd16_Rsp/1
  FeedbackModeStatAndRsp/54(StSrv_StMd17_Rsp) -> StSrv_StMd17_Rsp/1
  FeedbackModeStatAndRsp/55(StSrv_StMd18_Rsp) -> StSrv_StMd18_Rsp/1
  FeedbackModeStatAndRsp/56(StSrv_StMd19_Rsp) -> StSrv_StMd19_Rsp/1
  FeedbackModeStatAndRsp/57(StSrv_StMd20_Rsp) -> StSrv_StMd20_Rsp/1
  FeedbackModeStatAndRsp/58(StSrv_StMd21_Rsp) -> StSrv_StMd21_Rsp/1
  FeedbackModeStatAndRsp/59(StSrv_StMd22_Rsp) -> StSrv_StMd22_Rsp/1
  FeedbackModeStatAndRsp/60(StSrv_StMd23_Rsp) -> StSrv_StMd23_Rsp/1
  FeedbackModeStatAndRsp/61(StSrv_StMd24_Rsp) -> StSrv_StMd24_Rsp/1
  FeedbackModeStatAndRsp/62(StSrv_StMd25_Rsp) -> StSrv_StMd25_Rsp/1
  FeedbackModeStatAndRsp/63(StSrv_StMd26_Rsp) -> StSrv_StMd26_Rsp/1
  FeedbackModeStatAndRsp/64(StSrv_StMd27_Rsp) -> StSrv_StMd27_Rsp/1
  FeedbackModeStatAndRsp/65(StSrv_StMd28_Rsp) -> StSrv_StMd28_Rsp/1
  FeedbackModeStatAndRsp/66(StSrv_StMd29_Rsp) -> StSrv_StMd29_Rsp/1
  FeedbackModeStatAndRsp/67(StSrv_StMd30_Rsp) -> StSrv_StMd30_Rsp/1
  FeedbackModeStatAndRsp/68(StSrv_StMd31_Rsp) -> StSrv_StMd31_Rsp/1
  FeedbackModeStatAndRsp/69(StSrv_StMd32_Rsp) -> StSrv_StMd32_Rsp/1
  FeedbackModeStatAndRsp/70(HMI_2L_StMd1_Rsp) -> HMI_2L_StMd1_Rsp/1
  FeedbackModeStatAndRsp/71(HMI_2L_StMd2_Rsp) -> HMI_2L_StMd2_Rsp/1
  FeedbackModeStatAndRsp/72(HMI_2L_StMd3_Rsp) -> HMI_2L_StMd3_Rsp/1
  FeedbackModeStatAndRsp/73(HMI_2L_StMd4_Rsp) -> HMI_2L_StMd4_Rsp/1
  FeedbackModeStatAndRsp/74(HMI_2L_StMd5_Rsp) -> HMI_2L_StMd5_Rsp/1
  FeedbackModeStatAndRsp/75(HMI_2L_StMd6_Rsp) -> HMI_2L_StMd6_Rsp/1
  FeedbackModeStatAndRsp/76(HMI_2L_StMd7_Rsp) -> HMI_2L_StMd7_Rsp/1
  FeedbackModeStatAndRsp/77(HMI_2L_StMd8_Rsp) -> HMI_2L_StMd8_Rsp/1
  FeedbackModeStatAndRsp/78(HMI_2L_StMd9_Rsp) -> HMI_2L_StMd9_Rsp/1
  FeedbackModeStatAndRsp/79(HMI_2L_StMd10_Rsp) -> HMI_2L_StMd10_Rsp/1
  FeedbackModeStatAndRsp/80(HMI_2L_StMd11_Rsp) -> HMI_2L_StMd11_Rsp/1
  FeedbackModeStatAndRsp/81(HMI_2L_StMd12_Rsp) -> HMI_2L_StMd12_Rsp/1
  FeedbackModeStatAndRsp/82(HMI_2L_StMd13_Rsp) -> HMI_2L_StMd13_Rsp/1
  FeedbackModeStatAndRsp/83(HMI_2L_StMd14_Rsp) -> HMI_2L_StMd14_Rsp/1
  FeedbackModeStatAndRsp/84(HMI_2L_StMd15_Rsp) -> HMI_2L_StMd15_Rsp/1
  FeedbackModeStatAndRsp/85(HMI_2L_StMd16_Rsp) -> HMI_2L_StMd16_Rsp/1
  FeedbackModeStatAndRsp/86(HMI_2L_StMd17_Rsp) -> HMI_2L_StMd17_Rsp/1
  FeedbackModeStatAndRsp/87(HMI_2L_StMd18_Rsp) -> HMI_2L_StMd18_Rsp/1
  FeedbackModeStatAndRsp/88(HMI_2L_StMd19_Rsp) -> HMI_2L_StMd19_Rsp/1
  FeedbackModeStatAndRsp/89(HMI_2L_StMd20_Rsp) -> HMI_2L_StMd20_Rsp/1
  FeedbackModeStatAndRsp/90(HMI_2L_StMd21_Rsp) -> HMI_2L_StMd21_Rsp/1
  FeedbackModeStatAndRsp/91(HMI_2L_StMd22_Rsp) -> HMI_2L_StMd22_Rsp/1
  FeedbackModeStatAndRsp/92(HMI_2L_StMd23_Rsp) -> HMI_2L_StMd23_Rsp/1
  FeedbackModeStatAndRsp/93(HMI_2L_StMd24_Rsp) -> HMI_2L_StMd24_Rsp/1
  FeedbackModeStatAndRsp/94(HMI_2L_StMd25_Rsp) -> HMI_2L_StMd25_Rsp/1
  FeedbackModeStatAndRsp/95(HMI_2L_StMd26_Rsp) -> HMI_2L_StMd26_Rsp/1
  FeedbackModeStatAndRsp/96(HMI_2L_StMd27_Rsp) -> HMI_2L_StMd27_Rsp/1
  FeedbackModeStatAndRsp/97(HMI_2L_StMd28_Rsp) -> HMI_2L_StMd28_Rsp/1
  FeedbackModeStatAndRsp/98(HMI_2L_StMd29_Rsp) -> HMI_2L_StMd29_Rsp/1
  FeedbackModeStatAndRsp/99(HMI_2L_StMd30_Rsp) -> HMI_2L_StMd30_Rsp/1
  FeedbackModeStatAndRsp/100(HMI_2L_StMd31_Rsp) -> HMI_2L_StMd31_Rsp/1
  FeedbackModeStatAndRsp/101(HMI_2L_StMd32_Rsp) -> HMI_2L_StMd32_Rsp/1
  FeedbackModeStatAndRsp/102(HMI_2R_StMd1_Rsp) -> HMI_2R_StMd1_Rsp/1
  FeedbackModeStatAndRsp/103(HMI_2R_StMd2_Rsp) -> HMI_2R_StMd2_Rsp/1
  FeedbackModeStatAndRsp/104(HMI_2R_StMd3_Rsp) -> HMI_2R_StMd3_Rsp/1
  FeedbackModeStatAndRsp/105(HMI_2R_StMd4_Rsp) -> HMI_2R_StMd4_Rsp/1
  FeedbackModeStatAndRsp/106(HMI_2R_StMd5_Rsp) -> HMI_2R_StMd5_Rsp/1
  FeedbackModeStatAndRsp/107(HMI_2R_StMd6_Rsp) -> HMI_2R_StMd6_Rsp/1
  FeedbackModeStatAndRsp/108(HMI_2R_StMd7_Rsp) -> HMI_2R_StMd7_Rsp/1
  FeedbackModeStatAndRsp/109(HMI_2R_StMd8_Rsp) -> HMI_2R_StMd8_Rsp/1
  FeedbackModeStatAndRsp/110(HMI_2R_StMd9_Rsp) -> HMI_2R_StMd9_Rsp/1
  FeedbackModeStatAndRsp/111(HMI_2R_StMd10_Rsp) -> HMI_2R_StMd10_Rsp/1
  FeedbackModeStatAndRsp/112(HMI_2R_StMd11_Rsp) -> HMI_2R_StMd11_Rsp/1
  FeedbackModeStatAndRsp/113(HMI_2R_StMd12_Rsp) -> HMI_2R_StMd12_Rsp/1
  FeedbackModeStatAndRsp/114(HMI_2R_StMd13_Rsp) -> HMI_2R_StMd13_Rsp/1
  FeedbackModeStatAndRsp/115(HMI_2R_StMd14_Rsp) -> HMI_2R_StMd14_Rsp/1
  FeedbackModeStatAndRsp/116(HMI_2R_StMd15_Rsp) -> HMI_2R_StMd15_Rsp/1
  FeedbackModeStatAndRsp/117(HMI_2R_StMd16_Rsp) -> HMI_2R_StMd16_Rsp/1
  FeedbackModeStatAndRsp/118(HMI_2R_StMd17_Rsp) -> HMI_2R_StMd17_Rsp/1
  FeedbackModeStatAndRsp/119(HMI_2R_StMd18_Rsp) -> HMI_2R_StMd18_Rsp/1
  FeedbackModeStatAndRsp/120(HMI_2R_StMd19_Rsp) -> HMI_2R_StMd19_Rsp/1
  FeedbackModeStatAndRsp/121(HMI_2R_StMd20_Rsp) -> HMI_2R_StMd20_Rsp/1
  FeedbackModeStatAndRsp/122(HMI_2R_StMd21_Rsp) -> HMI_2R_StMd21_Rsp/1
  FeedbackModeStatAndRsp/123(HMI_2R_StMd22_Rsp) -> HMI_2R_StMd22_Rsp/1
  FeedbackModeStatAndRsp/124(HMI_2R_StMd23_Rsp) -> HMI_2R_StMd23_Rsp/1
  FeedbackModeStatAndRsp/125(HMI_2R_StMd24_Rsp) -> HMI_2R_StMd24_Rsp/1
  FeedbackModeStatAndRsp/126(HMI_2R_StMd25_Rsp) -> HMI_2R_StMd25_Rsp/1
  FeedbackModeStatAndRsp/127(HMI_2R_StMd26_Rsp) -> HMI_2R_StMd26_Rsp/1
  FeedbackModeStatAndRsp/128(HMI_2R_StMd27_Rsp) -> HMI_2R_StMd27_Rsp/1
  FeedbackModeStatAndRsp/129(HMI_2R_StMd28_Rsp) -> HMI_2R_StMd28_Rsp/1
  FeedbackModeStatAndRsp/130(HMI_2R_StMd29_Rsp) -> HMI_2R_StMd29_Rsp/1
  FeedbackModeStatAndRsp/131(HMI_2R_StMd30_Rsp) -> HMI_2R_StMd30_Rsp/1
  FeedbackModeStatAndRsp/132(HMI_2R_StMd31_Rsp) -> HMI_2R_StMd31_Rsp/1
  FeedbackModeStatAndRsp/133(HMI_2R_StMd32_Rsp) -> HMI_2R_StMd32_Rsp/1
  FeedbackModeStatAndRsp/134(StPassCmprtMd_Md1_CrtStat) -> StPassCmprtMd_Md1_CrtStat/1
  FeedbackModeStatAndRsp/135(StPassCmprtMd_Md2_CrtStat) -> StPassCmprtMd_Md2_CrtStat/1
  FeedbackModeStatAndRsp/136(StPassCmprtMd_Md3_CrtStat) -> StPassCmprtMd_Md3_CrtStat/1
  FeedbackModeStatAndRsp/137(StPassCmprtMd_Md4_CrtStat) -> StPassCmprtMd_Md4_CrtStat/1
  FeedbackModeStatAndRsp/138(StPassCmprtMd_Md5_CrtStat) -> StPassCmprtMd_Md5_CrtStat/1
  FeedbackModeStatAndRsp/139(StPassCmprtMd_Md6_CrtStat) -> StPassCmprtMd_Md6_CrtStat/1
  FeedbackModeStatAndRsp/140(StPassCmprtMd_Md7_CrtStat) -> StPassCmprtMd_Md7_CrtStat/1
  FeedbackModeStatAndRsp/141(StPassCmprtMd_Md8_CrtStat) -> StPassCmprtMd_Md8_CrtStat/1
  FeedbackModeStatAndRsp/142(StPassCmprtMd_Md9_CrtStat) -> StPassCmprtMd_Md9_CrtStat/1
  FeedbackModeStatAndRsp/143(StPassCmprtMd_Md10_CrtStat) -> StPassCmprtMd_Md10_CrtStat/1
  FeedbackModeStatAndRsp/144(StPassCmprtMd_Md11_CrtStat) -> StPassCmprtMd_Md11_CrtStat/1
  FeedbackModeStatAndRsp/145(StPassCmprtMd_Md12_CrtStat) -> StPassCmprtMd_Md12_CrtStat/1
  FeedbackModeStatAndRsp/146(StPassCmprtMd_Md13_CrtStat) -> StPassCmprtMd_Md13_CrtStat/1
  FeedbackModeStatAndRsp/147(StPassCmprtMd_Md14_CrtStat) -> StPassCmprtMd_Md14_CrtStat/1
  FeedbackModeStatAndRsp/148(StPassCmprtMd_Md15_CrtStat) -> StPassCmprtMd_Md15_CrtStat/1
  FeedbackModeStatAndRsp/149(StPassCmprtMd_Md16_CrtStat) -> StPassCmprtMd_Md16_CrtStat/1
  FeedbackModeStatAndRsp/150(StPassCmprtMd_Md17_CrtStat) -> StPassCmprtMd_Md17_CrtStat/1
  FeedbackModeStatAndRsp/151(StPassCmprtMd_Md18_CrtStat) -> StPassCmprtMd_Md18_CrtStat/1
  FeedbackModeStatAndRsp/152(StPassCmprtMd_Md19_CrtStat) -> StPassCmprtMd_Md19_CrtStat/1
  FeedbackModeStatAndRsp/153(StPassCmprtMd_Md20_CrtStat) -> StPassCmprtMd_Md20_CrtStat/1
  FeedbackModeStatAndRsp/154(StPassCmprtMd_Md21_CrtStat) -> StPassCmprtMd_Md21_CrtStat/1
  FeedbackModeStatAndRsp/155(StPassCmprtMd_Md22_CrtStat) -> StPassCmprtMd_Md22_CrtStat/1
  FeedbackModeStatAndRsp/156(StPassCmprtMd_Md23_CrtStat) -> StPassCmprtMd_Md23_CrtStat/1
  FeedbackModeStatAndRsp/157(StPassCmprtMd_Md24_CrtStat) -> StPassCmprtMd_Md24_CrtStat/1
  FeedbackModeStatAndRsp/158(StPassCmprtMd_Md25_CrtStat) -> StPassCmprtMd_Md25_CrtStat/1
  FeedbackModeStatAndRsp/159(StPassCmprtMd_Md26_CrtStat) -> StPassCmprtMd_Md26_CrtStat/1
  FeedbackModeStatAndRsp/160(StPassCmprtMd_Md27_CrtStat) -> StPassCmprtMd_Md27_CrtStat/1
  FeedbackModeStatAndRsp/161(StPassCmprtMd_Md28_CrtStat) -> StPassCmprtMd_Md28_CrtStat/1
  FeedbackModeStatAndRsp/162(StPassCmprtMd_Md29_CrtStat) -> StPassCmprtMd_Md29_CrtStat/1
  FeedbackModeStatAndRsp/163(StPassCmprtMd_Md30_CrtStat) -> StPassCmprtMd_Md30_CrtStat/1
  FeedbackModeStatAndRsp/164(StPassCmprtMd_Md31_CrtStat) -> StPassCmprtMd_Md31_CrtStat/1
  FeedbackModeStatAndRsp/165(StPassCmprtMd_Md32_CrtStat) -> StPassCmprtMd_Md32_CrtStat/1
  FeedbackModeStatAndRsp/166(SRSCrt_MdSw1_Stat_67_2) -> Data Type Conversion/1
  FeedbackModeStatAndRsp/167(SRSCrt_MdSw2_Stat_67_2) -> Data Type Conversion1/1
  FeedbackModeStatAndRsp/168(SRSCrt_MdSw3_Stat_67_2) -> Data Type Conversion2/1
  FeedbackModeStatAndRsp/169(SRSCrt_MdSw4_Stat_67_2) -> Data Type Conversion3/1
  FeedbackModeStatAndRsp/170(SRSCrt_MdSw5_Stat_67_2) -> Data Type Conversion4/1
  FeedbackModeStatAndRsp/171(SRSCrt_MdSw6_Stat_67_2) -> Data Type Conversion5/1
  FeedbackModeStatAndRsp/172(SRSCrt_MdSw7_Stat_67_2) -> Data Type Conversion6/1
  FeedbackModeStatAndRsp/173(SRSCrt_MdSw8_Stat_67_2) -> Data Type Conversion7/1
  FeedbackModeStatAndRsp/174(SRSCrt_MdSw9_Stat_67_2) -> Data Type Conversion8/1
  FeedbackModeStatAndRsp/175(SRSCrt_MdSw10_Stat_67_2) -> Data Type Conversion9/1
  [LfVipArrivedAtTargetPos] -> AND/1
  [RtVipArrivedAtTargetPos] -> AND/2
  [isLfLugArrivedAtTargetPos] -> AND1/1
  [isRtLugArrivedAtTargetPos] -> AND1/2
  SwIntRtLy_Val_read/1 -> Subsystem/78(SwIntRtLy)
  SwIntLfFamly_Val_read/1 -> Subsystem/75(SwIntLfFamly)
  SwIntINTM_Val_read/1 -> Subsystem/74(SwIntINTM)
  SoftIntLfLy_Val_read/1 -> Subsystem/71(SoftIntLfLy)
  SoftIntRtLy_Val_read/1 -> Subsystem/73(SoftIntRtLy)
  SwIntRtFamly_Val_read/1 -> Subsystem/77(SwIntRtFamly)
  SoftIntLfFamly_Val_read/1 -> Subsystem/70(SoftIntLfFamly)
  SoftIntRtFamly_Val_read/1 -> Subsystem/72(SoftIntRtFamly)
  SwIntLfLy_Val_read/1 -> Subsystem/76(SwIntLfLy)
  SoftIntINTM_Val_read/1 -> Subsystem/69(SoftIntINTM)
  isINTMDoneOK/1 -> Subsystem/79(isINTMDoneOK)
  isFamlyLDoneOK/1 -> Subsystem/80(isFamlyLDoneOK)
  isFamlyRDoneOK/1 -> Subsystem/81(isFamlyRDoneOK)
  isLfLyDoneOK/1 -> Subsystem/82(isLfLyDoneOK)
  isRtLyDoneOK/1 -> Subsystem/83(isRtLyDoneOK)
  isINTMDoneFailed/1 -> Subsystem/84(isINTMDoneFailed)
  isFamlyLDoneFailed/1 -> Subsystem/85(isFamlyLDoneFailed)
  isFamlyRDoneFailed/1 -> Subsystem/86(isFamlyRDoneFailed)
  isLfLyDoneFailed/1 -> Subsystem/87(isLfLyDoneFailed)
  isRtLyDoneFailed/1 -> Subsystem/88(isRtLyDoneFailed)
  SRSModeCheck/1(SRSModeState) -> SRSMode/1
  [MdStateBus] -> SRSModeCheck/1(MdStatusBus)
  [MdSrcTp] -> SRSModeCheck/2(MdSrcTp)
  PosArray_Val_read/1 -> FeedbackModeStatAndRsp/9(PosArray_Val_read)
  Data Type Conversion/1 -> SRSCrt_MdSw1_Stat_67_2/1
  Data Type Conversion1/1 -> SRSCrt_MdSw2_Stat_67_2/1
  Data Type Conversion2/1 -> SRSCrt_MdSw3_Stat_67_2/1
  Data Type Conversion3/1 -> SRSCrt_MdSw4_Stat_67_2/1
  Data Type Conversion4/1 -> SRSCrt_MdSw5_Stat_67_2/1
  Data Type Conversion5/1 -> SRSCrt_MdSw6_Stat_67_2/1
  Data Type Conversion6/1 -> SRSCrt_MdSw7_Stat_67_2/1
  Data Type Conversion7/1 -> SRSCrt_MdSw8_Stat_67_2/1
  Data Type Conversion8/1 -> SRSCrt_MdSw9_Stat_67_2/1
  Data Type Conversion9/1 -> SRSCrt_MdSw10_Stat_67_2/1
  INTMMdReq_Val_read/1 -> Subsystem/59(INTMMdReq)
  LfFamlyReq_Val_read/1 -> Subsystem/60(LfFamlyReq)
  LfLyMdReq_Val_read/1 -> Subsystem/61(LfLyMdReq)
  RtFamlyMdReq_Val_read/1 -> Subsystem/62(RtFamlyMdReq)
  RtLyMdReq_Val_read/1 -> Subsystem/63(RtLyMdReq)
  INTMSrcReqTp_Val_read/1 -> Subsystem/64(INTMSrcReqTp)
  LfFamlySrcReqTp_Val_read/1 -> Subsystem/65(LfFamlySrcReqTp)
  LfLySrcReqTp_Val_read/1 -> Subsystem/66(LfLySrcReqTp)
  RtFamlySrcReqTp_Val_read/1 -> Subsystem/67(RtFamlySrcReqTp)
  RtLySrcReqTp_Val_read/1 -> Subsystem/68(RtLySrcReqTp)
  AllVipSrcReqTp_Val_read/1 -> Subsystem/89(AllVipSrcReqTp)
  LugMdLtAvl_Val_read/1 -> Subsystem/90(LugMdLtAvl_Val_read)
  LugMdRtAvl_Val_read/1 -> Subsystem/91(LugMdRtAvl_Val_read)
  VipMdLtAvl_Val_read/1 -> Subsystem/92(VipMdLtAvl_Val_read)
  VipMdRtAvl_Val_read/1 -> Subsystem/93(VipMdRtAvl_Val_read)
  SwIntAllVip_Val_read/1 -> Subsystem/94(SwIntAllVip)
  IntimacyRtMdSrcTp_Val_read/1 -> Subsystem/96(IntimacyRtMdSrcTp_Val_read)
  IntimacyRtMdReq_Val_read/1 -> Subsystem/95(IntimacyRtMdReq_Val_read)
  isINTMRDoneFailed_Val_read/1 -> Subsystem/97(isINTMRDoneFailed_Val_read)
  isINTMRDoneOK_Val_read/1 -> Subsystem/98(isINTMRDoneOK_Val_read)
  isLgrstCloseLDoneFailed_Val_read/1 -> Subsystem/99(isLgrstCloseLDoneFailed_Val_read)
  isLgrstCloseLDoneOK_Val_read/1 -> Subsystem/100(isLgrstCloseLDoneOK_Val_read)
  isLgrstCloseRDoneFailed_Val_read/1 -> Subsystem/101(isLgrstCloseRDoneFailed_Val_read)
  isLgrstCloseRDoneOK_Val_read/1 -> Subsystem/102(isLgrstCloseRDoneOK_Val_read)
  isLgrstOpenLDoneFailed_Val_read/1 -> Subsystem/103(isLgrstOpenLDoneFailed_Val_read)
  isLgrstOpenLDoneOK_Val_read/1 -> Subsystem/104(isLgrstOpenLDoneOK_Val_read)
  isLgrstOpenRDoneFailed_Val_read/1 -> Subsystem/105(isLgrstOpenRDoneFailed_Val_read)
  isLgrstOpenRDoneOK_Val_read/1 -> Subsystem/106(isLgrstOpenRDoneOK_Val_read)
  LgrstCloseLtMdReq_Val_read/1 -> Subsystem/107(LgrstCloseLtMdReq_Val_read)
  LgrstCloseLtSrcReqTp_Val_read/1 -> Subsystem/108(LgrstCloseLtSrcReqTp_Val_read)
  LgrstCloseRtMdReq_Val_read/1 -> Subsystem/109(LgrstCloseRtMdReq_Val_read)
  LgrstCloseRtSrcReqTp_Val_read/1 -> Subsystem/110(LgrstCloseRtSrcReqTp_Val_read)
  LgrstOpenLtMdReq_Val_read/1 -> Subsystem/111(LgrstOpenLtMdReq_Val_read)
  LgrstOpenLtSrcReqTp_Val_read/1 -> Subsystem/112(LgrstOpenLtSrcReqTp_Val_read)
  LgrstOpenRtMdReq_Val_read/1 -> Subsystem/113(LgrstOpenRtMdReq_Val_read)
  LgrstOpenRtSrcReqTp_Val_read/1 -> Subsystem/114(LgrstOpenRtSrcReqTp_Val_read)
  SoftIntIntimacyRt_Val_read/1 -> Subsystem/115(SoftIntIntimacyRt_Val_read)
  SoftIntLgrstCloseLt_Val_read/1 -> Subsystem/116(SoftIntLgrstCloseLt_Val_read)
  SoftIntLgrstCloseRt_Val_read/1 -> Subsystem/117(SoftIntLgrstCloseRt_Val_read)
  SoftIntLgrstOpenLt_Val_read/1 -> Subsystem/118(SoftIntLgrstOpenLt_Val_read)
  SoftIntLgrstOpenRt_Val_read/1 -> Subsystem/119(SoftIntLgrstOpenRt_Val_read)
  SwIntIntimacyRt_Val_read/1 -> Subsystem/120(SwIntIntimacyRt_Val_read)
  SwIntLgrstCloseLt_Val_read/1 -> Subsystem/121(SwIntLgrstCloseLt_Val_read)
  SwIntLgrstCloseRt_Val_read/1 -> Subsystem/122(SwIntLgrstCloseRt_Val_read)
  SwIntLgrstOpenLt_Val_read/1 -> Subsystem/123(SwIntLgrstOpenLt_Val_read)
  SwIntLgrstOpenRt_Val_read/1 -> Subsystem/124(SwIntLgrstOpenRt_Val_read)
  [MdTrgtPos] -> FeedbackModeStatAndRsp/6(isArrivedAtTargetPos)
  [MdSrcTp] -> FeedbackModeStatAndRsp/7(ModeSrcTp)
  [MdRsp] -> FeedbackModeStatAndRsp/8(ModeRsp)
  [MdBsy] -> FeedbackModeStatAndRsp/10(MdExit)
  Subsystem/4(MdStateBus) -> [MdStateBus]
  Subsystem/5(MdBsy) -> [MdBsy]
  Subsystem/6(MdSrcTp) -> [MdSrcTp]  "MdSrcTp"
  Subsystem/7(MdRsp) -> [MdRsp]
